simulink model "DreiTankSim_Visual"  (R2021a)
settings: Solver=ode5  StartTime=0.0  StopTime=inf  RelTol=1e-3
model workspace (MAT data in the model file):
  A1 = 20
  A2 = 20
  A3 = 20
  Kt = 1
  Kv = 8.75529661017
  Kvgekop = 6.21621117085
  k1 = 1.5
  k2 = 1.5
  k3 = 1.5
  k4 = 5
  k5 = 5
  k6 = 5
libraries: pid_lib x3, sldrtlib x3
(part 1 of 2)
settings Model: Creator=Ogulcan  LastModifiedBy=Ogulcan
settings RTWCC: Description=Simulink Desktop Real-Time  SystemTargetFile=sldrt.tlc  TemplateMakefile=sldrt.tmf  RTWCompilerOptimization=on
settings CodeAppCC: MaxIdLength=95
settings SimulinkDesktopRealTimeCC: TargetPreCompLibLocation=E:\MathWorks\r2021a\toolbox\sldrt\lib\win64

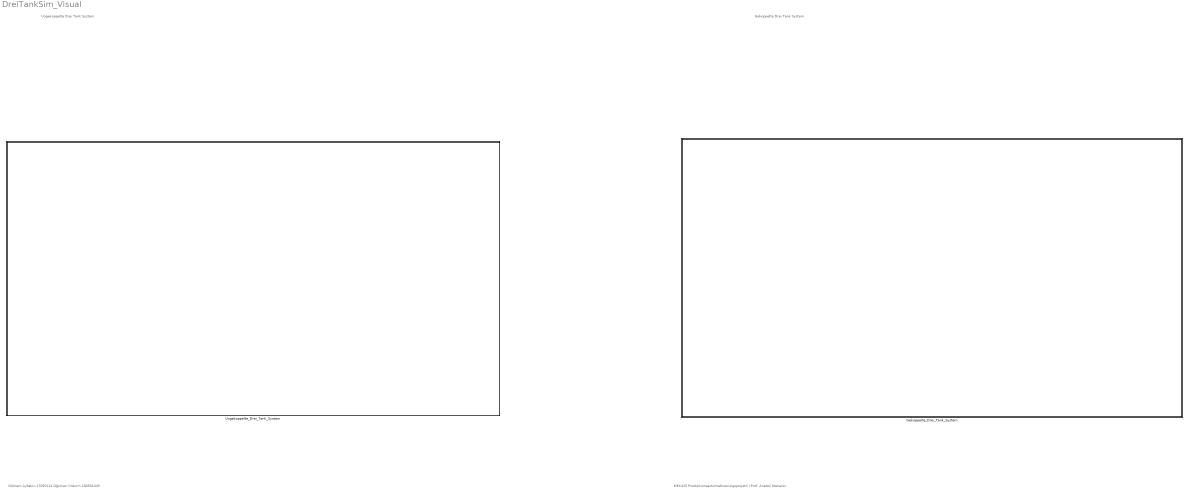
== system DreiTankSim_Visual ==
  note: Görkem Aytekin 17050114
      | Oğulcan Yıldırım 180501045
  note: Ungekoppelte Drei Tank System
  note: Gekoppelte Drei Tank System
  note: MEC425 Produktionsautomatisierungsprojekt I Prof. Anatoli Makarov
  Gekoppelte_Drei_Tank_System : Subsystem
      mask Display: image('C:\Users\Oğulcan\OneDrive\Masaüstü\GörOgiProjekt\MatlabGUİ\GuiTemiz\GekoppeltSim.png'); % Use "Edit Image" on toolstrip to change.
  Ungekoppelte_Drei_Tank_System : Subsystem
      mask Display: image('C:\Users\Oğulcan\OneDrive\Masaüstü\GörOgiProjekt\MatlabGUİ\GuiTemiz\ungekoppeltFotoSim.png'); % Use "Edit Image" on toolstrip to change.

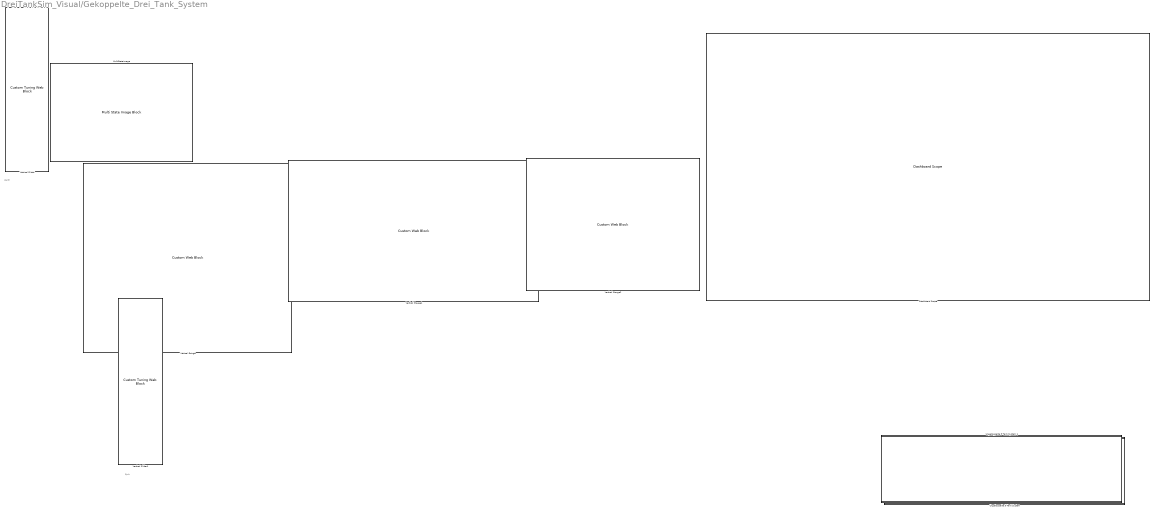
== system DreiTankSim_Visual/Gekoppelte_Drei_Tank_System ==
  note: Quit
  note: Ventil
  Dashboard Scope : DashboardScope  Ymin=0  Ymax=5000  LegendPosition=Right
  MultiStateImage : MultiStateImageBlock  ScaleMode=Fill
  "Ungekoppelte 3 Tank System " : Subsystem
      mask Display: image('C:\Users\Oğulcan\OneDrive\Masaüstü\GörOgiProjekt\MatlabGUİ\GuiTemiz\Taulogo.png'); % Use "Edit Image" on toolstrip to change.
  Ungekoppelte 3 Tank System 1 : Subsystem
      mask Display: image('C:\Users\Oğulcan\OneDrive\Masaüstü\GörOgiProjekt\MatlabGUİ\GuiTemiz\Taulogo.png'); % Use "Edit Image" on toolstrip to change.
  Vertical Gauge : CustomWebBlock  LabelPosition=Hide  ShowInitialText=on  Configuration="{\"components\":[{\"name\":\"LinearScaleComponent\",\"settings\":{\"bounds\":{\"max\":5000,\"min\":0,\"tickInterval\":500},\"internalTickHeightScaleFactor\":0.5,\"labelColor\":[0,255,0],\"labelFont\":{\"font\":\"Arial\",\"fontSize\":12},\"labelTransparency\":0.5,\"needleImage\":{\"size\":[21,75],\"src\":\"data:image\\/svg+xml;base64,PHN2ZyB4bWxucz0iaHR0cDovL3d3dy53My5vcmcvMjAwMC9zdmciIHhtbG5zOnhsaW5rPSJodHRwOi8vd3d3LnczLm9yZy8xOTk5L3hsaW5rIiB2aWV3Qm94PSIwIDAgMjEgNzUiPjxkZWZzPjxzdHlsZT4uY2xzLTF7ZmlsbDpub25lO30uY2xzLTJ7aXNvbGF0aW9uOmlzb2xhdGU7fS5jbHMtM3tjbGlwLXBhdGg6dXJsKCNjbGlwLXBhdGgpO30uY2xzLTR7b3BhY2l0eTowLjM7bWl4LWJsZW5kLW1vZGU6bXVsdGlwbHk7fS5jbHMtNXtmaWxsOiNlYjI2Mjk7fTwvc3R5bGU+PGNsaXBQYXRoIGlkPSJjbGlwLXBhdGgiIHRyYW5zZm9y ...(+1928 chars)\",\"srcOrientation\":\"horizontal\"},\"needleOffset\":[-0.01094391244870041,0],\"needleSize\":{\"height\":0.06,\"width\":0.48},\"position\":[-0.022724338282763074,0.21281719924812031,0.4357377819548872,0.6807617817947063],\"scaleColors\":[],\"scaleColorsSize\":0.2,\"showLabels\":1,\"showMinorTicks\":0,\"showSpanLine\":1,\"showTicks\":1,\"tickColor\":[204,204,204],\"tickTransparency\":0.5,\"valueBarColor\":[127,205,255],\"valueBarOffset\":-0.01,\"valueBarSize\":0.92,\"valueBarTransparency\":1}},{\"name\":\"BackgroundImageComponent\",\"settings\":{\"image\":{\"size\":[293,266],\"src\":\"data:image\\/png;base64,iVBORw0KGgoAAAANSUhEUgAAASUAAAEKCAYAAABUnUOUAAAACXBIWXMAABJ0AAASdAHeZh94AAANmUlEQVR4Xu3djVLbWBIGUP8Qktr3f9cEMPbeNhYjPBDEYMzt24eq1CSzxHSfT\\/6Qxay1WvmYBPbtN4f2a79er4\\/\\/RDOWwH4f0a4fp5xn\\/xxr0eTbbJLP\\/+nx40A9e5DzP3\\/6a3iAPgQ2m018s5k+5NxHLP+aonwpdZqLsb5I4HA4KKMvsr3Uw5YvpbPvnpdy9TiJBF45W040\\/Xijli+liNRBOd6B\\/dpGcs6Rs1LKkZMpLyDw1ks3L+kugHvBh1BKF8T0UAQIfF5AKX3e0CMQIHBBAaXUMF3svuAR1fFDxX9\\/dvpv0F ...(+4502 chars)\",\"srcOrientation\":\"vertical\"},\"position\":[0,0,1,1],\"scaleMode\":\"0\"}},{\"name\":\"ForegroundImageComponent\",\"settings\":{\"image\":{\"size\":[0,0],\"src\":\"default\",\"srcOrientation\":[]},\"isForeground\":1,\"position\":[0,0,1,1],\"scaleMode\":\"0\"}}],\"settings\":{\"BindingType\":\"signal\",\"backgroundColor\":[255,255,255,\"1\"],\"backgroundOffset\":0,\"backgroundOpacity\":0,\"fixedAspectRatio\":\"on\",\"orientation\":\"vertical\",\"showBackgroundColor\":false,\"value\":0},\"type\":\"LinearGauge\"}"
  Vertical Gauge1 : CustomWebBlock  LabelPosition=Hide  ShowInitialText=on  Configuration="{\"components\":[{\"name\":\"LinearScaleComponent\",\"settings\":{\"bounds\":{\"max\":5000,\"min\":0,\"tickInterval\":500},\"internalTickHeightScaleFactor\":0.5,\"labelColor\":[0,255,0],\"labelFont\":{\"font\":\"Arial\",\"fontSize\":12},\"labelTransparency\":0.5,\"needleImage\":{\"size\":[21,75],\"src\":\"data:image\\/svg+xml;base64,PHN2ZyB4bWxucz0iaHR0cDovL3d3dy53My5vcmcvMjAwMC9zdmciIHhtbG5zOnhsaW5rPSJodHRwOi8vd3d3LnczLm9yZy8xOTk5L3hsaW5rIiB2aWV3Qm94PSIwIDAgMjEgNzUiPjxkZWZzPjxzdHlsZT4uY2xzLTF7ZmlsbDpub25lO30uY2xzLTJ7aXNvbGF0aW9uOmlzb2xhdGU7fS5jbHMtM3tjbGlwLXBhdGg6dXJsKCNjbGlwLXBhdGgpO30uY2xzLTR7b3BhY2l0eTowLjM7bWl4LWJsZW5kLW1vZGU6bXVsdGlwbHk7fS5jbHMtNXtmaWxsOiNlYjI2Mjk7fTwvc3R5bGU+PGNsaXBQYXRoIGlkPSJjbGlwLXBhdGgiIHRyYW5zZm9y ...(+1928 chars)\",\"srcOrientation\":\"horizontal\"},\"needleOffset\":[-0.01094391244870041,0],\"needleSize\":{\"height\":0.06,\"width\":0.38},\"position\":[-0.05307664627563872,0.23195564516129033,0.3876008064516129,0.9625764663548039],\"scaleColors\":[],\"scaleColorsSize\":0.2,\"showLabels\":1,\"showMinorTicks\":0,\"showSpanLine\":1,\"showTicks\":1,\"tickColor\":[204,204,204],\"tickTransparency\":0.5,\"valueBarColor\":[127,205,255],\"valueBarOffset\":-0.03,\"valueBarSize\":0.92,\"valueBarTransparency\":1}},{\"name\":\"BackgroundImageComponent\",\"settings\":{\"image\":{\"size\":[313,175],\"src\":\"data:image\\/png;base64,iVBORw0KGgoAAAANSUhEUgAAATkAAACvCAYAAACGqakbAAAACXBIWXMAABJ0AAASdAHeZh94AAAG3ElEQVR4Xu3dwXIbRwwFwCiV\\/\\/\\/gHKyYPim0E3mWGDyspnVTFQfANshHSjLptz98rQq8Px14fP\\/nahG3jwt8+z7B24cp7DG+kj0DeHC+7vrxgfJ6NRUIECgVEHKlnIrdSOD5ycmT1Y2WtzKqkFvRctuvLPD8a4ivfK1HXZuQO2rdLpbAeQJC7rydu2ICRwkIuaPW7WIJnCcg5M7buSsmcJSAkDtq3S6WwHkCQu68nbtiAkcJCLmj1u1iCZwnIOTO27krJnCUgJB7fd3+EenrhioQ2CYg5LbRKkyAwAQBITdhC2YgQGCbgJDbRqvw ...(+2096 chars)\",\"srcOrientation\":\"vertical\"},\"position\":[0,0,1,1],\"scaleMode\":\"0\"}},{\"name\":\"ForegroundImageComponent\",\"settings\":{\"image\":{\"size\":[0,0],\"src\":\"default\",\"srcOrientation\":[]},\"isForeground\":1,\"position\":[0,0,1,1],\"scaleMode\":\"0\"}}],\"settings\":{\"BindingType\":\"signal\",\"backgroundColor\":[255,255,255,\"1\"],\"backgroundOffset\":0,\"backgroundOpacity\":0,\"fixedAspectRatio\":\"on\",\"orientation\":\"vertical\",\"showBackgroundColor\":false,\"value\":0},\"type\":\"LinearGauge\"}"
  Vertical Gauge2 : CustomWebBlock  LabelPosition=Hide  ShowInitialText=on  Configuration="{\"components\":[{\"name\":\"LinearScaleComponent\",\"settings\":{\"bounds\":{\"max\":5000,\"min\":0,\"tickInterval\":500},\"internalTickHeightScaleFactor\":0.5,\"labelColor\":[0,255,0],\"labelFont\":{\"font\":\"Arial\",\"fontSize\":12},\"labelTransparency\":0.5,\"needleImage\":{\"size\":[21,75],\"src\":\"data:image\\/svg+xml;base64,PHN2ZyB4bWxucz0iaHR0cDovL3d3dy53My5vcmcvMjAwMC9zdmciIHhtbG5zOnhsaW5rPSJodHRwOi8vd3d3LnczLm9yZy8xOTk5L3hsaW5rIiB2aWV3Qm94PSIwIDAgMjEgNzUiPjxkZWZzPjxzdHlsZT4uY2xzLTF7ZmlsbDpub25lO30uY2xzLTJ7aXNvbGF0aW9uOmlzb2xhdGU7fS5jbHMtM3tjbGlwLXBhdGg6dXJsKCNjbGlwLXBhdGgpO30uY2xzLTR7b3BhY2l0eTowLjM7bWl4LWJsZW5kLW1vZGU6bXVsdGlwbHk7fS5jbHMtNXtmaWxsOiNlYjI2Mjk7fTwvc3R5bGU+PGNsaXBQYXRoIGlkPSJjbGlwLXBhdGgiIHRyYW5zZm9y ...(+1928 chars)\",\"srcOrientation\":\"horizontal\"},\"needleOffset\":[-0.01094391244870041,0],\"needleSize\":{\"height\":0.06,\"width\":0.48},\"position\":[0.003223915592028136,0.4366930751173709,0.5352112676056338,0.9722547870261821],\"scaleColors\":[],\"scaleColorsSize\":0.2,\"showLabels\":1,\"showMinorTicks\":0,\"showSpanLine\":1,\"showTicks\":1,\"tickColor\":[204,204,204],\"tickTransparency\":0.5,\"valueBarColor\":[127,205,255],\"valueBarOffset\":-0.01,\"valueBarSize\":0.91,\"valueBarTransparency\":1}},{\"name\":\"BackgroundImageComponent\",\"settings\":{\"image\":{\"size\":[235,176],\"src\":\"data:image\\/png;base64,iVBORw0KGgoAAAANSUhEUgAAAOsAAACwCAYAAADuQ5nhAAAG4klEQVR4Xu3d7U5aWwAGYfmw3v\\/F+kMpcNaiajytRa2V4vCQGKNR2e8M44Ym3V5duSGAAAIIIIAAAggggAACCCCAAAIfILDb7Rbz7QM\\/wrd+DQK75XL5fRzq7mscrqP8H4HNZjP8LTdT4GKxmCLdmgS2D5Huh+f5Nj92+0oEZqir1WrG+iiQxK8k8A3Hut1ul4+hrtfr\\/XTt7PoGcGf4JfMp0f7m5uYg0W\\/cMzT0dw5pPnN6DHX\\/8HT46Sd7DfR3IH\\/2T5mxPnc1hc7fxG4tAkc9E96SbU2YgFjDck1rERBry6c1YQJiDcs1rUVArC2f1oQJiDUs17QWAbG2fFoT ...(+2100 chars)\",\"srcOrientation\":\"vertical\"},\"position\":[0,0,1,1],\"scaleMode\":\"0\"}},{\"name\":\"ForegroundImageComponent\",\"settings\":{\"image\":{\"size\":[0,0],\"src\":\"default\",\"srcOrientation\":[]},\"isForeground\":1,\"position\":[0,0,1,1],\"scaleMode\":\"0\"}}],\"settings\":{\"BindingType\":\"signal\",\"backgroundColor\":[255,255,255,\"1\"],\"backgroundOffset\":0,\"backgroundOpacity\":0,\"fixedAspectRatio\":\"on\",\"orientation\":\"vertical\",\"showBackgroundColor\":false,\"value\":0},\"type\":\"LinearGauge\"}"
  Vertical Slider : CustomTuningWebBlock  LabelPosition=Hide  ShowInitialText=on  Configuration="{\"components\":[{\"name\":\"LinearScaleComponent\",\"settings\":{\"bounds\":{\"max\":10,\"min\":0,\"tickInterval\":\"auto\"},\"internalTickHeightScaleFactor\":1,\"labelColor\":[255,255,0],\"labelFont\":{\"font\":\"Arial\",\"fontSize\":12},\"labelOffset\":0.05,\"labelTransparency\":1,\"needleImage\":{\"size\":[842,596],\"src\":\"data:image\\/svg+xml;base64,PD94bWwgdmVyc2lvbj0iMS4wIiBlbmNvZGluZz0idXRmLTgiPz4NCjwhLS0gR2VuZXJhdG9yOiBBZG9iZSBJbGx1c3RyYXRvciAyNS4wLjAsIFNWRyBFeHBvcnQgUGx1Zy1JbiAuIFNWRyBWZXJzaW9uOiA2LjAwIEJ1aWxkIDApICAtLT4NCjxzdmcgdmVyc2lvbj0iMS4xIg0KCSBpZD0ic3ZnOCIgeG1sbnM6Y2M9Imh0dHA6Ly9jcmVhdGl2ZWNvbW1vbnMub3JnL25zIyIgeG1sbnM6ZGM9Imh0dHA6Ly9wdXJsLm9yZy9kYy9lbGVtZW50cy8xLjEvIiB4bWxuczppbmtzY2FwZT0iaHR0cDovL3d3dy5pbmtzY2FwZS5vcmcvbmFtZXNw ...(+2376 chars)\",\"srcOrientation\":\"vertical\"},\"needleOffset\":[0.02,-0.8],\"needleSize\":{\"height\":0.07532387955182072,\"width\":0.43386243386243384},\"position\":[0.027412280701754384,0.2830188679245283,0.5832841981132075,0.9524201127819549],\"scaleColors\":[],\"scaleColorsSize\":0.2,\"showLabels\":1,\"showMinorTicks\":0,\"showSpanLine\":1,\"showTicks\":1,\"tickColor\":[234,234,234],\"tickTransparency\":1,\"valueBarColor\":[0,255,255],\"valueBarOffset\":-0.28,\"valueBarSize\":0.1,\"valueBarTransparency\":1}},{\"name\":\"BackgroundImageComponent\",\"settings\":{\"image\":{\"size\":[101,380],\"src\":\"data:image\\/svg+xml;base64,PD94bWwgdmVyc2lvbj0iMS4wIiBlbmNvZGluZz0iVVRGLTgiIHN0YW5kYWxvbmU9Im5vIj8+CjxzdmcKICAgeG1sbnM6ZGM9Imh0dHA6Ly9wdXJsLm9yZy9kYy9lbGVtZW50cy8xLjEvIgogICB4bWxuczpjYz0iaHR0cDovL2NyZWF0aXZlY29tbW9ucy5vcmcvbnMjIgogICB4bWxuczpyZGY9Imh0dHA6Ly93d3cudzMub3JnLzE5OTkvMDIvMjItcmRmLXN5bnRheC1ucyMiCiAgIHhtbG5zOnN2Zz0iaHR0cDovL3d3dy53My5vcmcvMjAwMC9zdmciCiAgIHhtbG5zPSJodHRwOi8vd3d3LnczLm9yZy8yMDAwL3N2ZyIKICAgeG1sbnM6 ...(+3116 chars)\",\"srcOrientation\":\"vertical\"},\"position\":[0,0,1,1],\"scaleMode\":\"0\"}},{\"name\":\"ForegroundImageComponent\",\"settings\":{\"image\":{\"size\":[0,0],\"src\":\"default\",\"srcOrientation\":[]},\"isForeground\":1,\"position\":[0,0,1,1],\"scaleMode\":\"0\"}}],\"settings\":{\"BindingType\":\"param\",\"aspectRatio\":0.2651006711409396,\"backgroundColor\":[0,0,0,\"1\"],\"backgroundOffset\":0,\"backgroundOpacity\":1,\"fixedAspectRatio\":\"on\",\"orientation\":\"vertical\",\"showBackgroundColor\":false,\"value\":0},\"type\":\"LinearGauge\"}"
  Vertical Slider1 : CustomTuningWebBlock  LabelPosition=Hide  ShowInitialText=on  Configuration="{\"components\":[{\"name\":\"LinearScaleComponent\",\"settings\":{\"bounds\":{\"max\":2,\"min\":0,\"tickInterval\":\"auto\"},\"internalTickHeightScaleFactor\":1,\"labelColor\":[255,255,0],\"labelFont\":{\"font\":\"Arial\",\"fontSize\":12},\"labelOffset\":0.05,\"labelTransparency\":1,\"needleImage\":{\"size\":[842,596],\"src\":\"data:image\\/svg+xml;base64,PD94bWwgdmVyc2lvbj0iMS4wIiBlbmNvZGluZz0idXRmLTgiPz4NCjwhLS0gR2VuZXJhdG9yOiBBZG9iZSBJbGx1c3RyYXRvciAyNS4wLjAsIFNWRyBFeHBvcnQgUGx1Zy1JbiAuIFNWRyBWZXJzaW9uOiA2LjAwIEJ1aWxkIDApICAtLT4NCjxzdmcgdmVyc2lvbj0iMS4xIg0KCSBpZD0ic3ZnOCIgeG1sbnM6Y2M9Imh0dHA6Ly9jcmVhdGl2ZWNvbW1vbnMub3JnL25zIyIgeG1sbnM6ZGM9Imh0dHA6Ly9wdXJsLm9yZy9kYy9lbGVtZW50cy8xLjEvIiB4bWxuczppbmtzY2FwZT0iaHR0cDovL3d3dy5pbmtzY2FwZS5vcmcvbmFtZXNw ...(+2376 chars)\",\"srcOrientation\":\"vertical\"},\"needleOffset\":[0.02,-0.8],\"needleSize\":{\"height\":0.07532387955182072,\"width\":0.43386243386243384},\"position\":[0.027412280701754384,0.2830188679245283,0.5832841981132075,0.9524201127819549],\"scaleColors\":[],\"scaleColorsSize\":0.2,\"showLabels\":1,\"showMinorTicks\":0,\"showSpanLine\":1,\"showTicks\":1,\"tickColor\":[234,234,234],\"tickTransparency\":1,\"valueBarColor\":[0,255,255],\"valueBarOffset\":-0.28,\"valueBarSize\":0.1,\"valueBarTransparency\":1}},{\"name\":\"BackgroundImageComponent\",\"settings\":{\"image\":{\"size\":[101,380],\"src\":\"data:image\\/svg+xml;base64,PD94bWwgdmVyc2lvbj0iMS4wIiBlbmNvZGluZz0iVVRGLTgiIHN0YW5kYWxvbmU9Im5vIj8+CjxzdmcKICAgeG1sbnM6ZGM9Imh0dHA6Ly9wdXJsLm9yZy9kYy9lbGVtZW50cy8xLjEvIgogICB4bWxuczpjYz0iaHR0cDovL2NyZWF0aXZlY29tbW9ucy5vcmcvbnMjIgogICB4bWxuczpyZGY9Imh0dHA6Ly93d3cudzMub3JnLzE5OTkvMDIvMjItcmRmLXN5bnRheC1ucyMiCiAgIHhtbG5zOnN2Zz0iaHR0cDovL3d3dy53My5vcmcvMjAwMC9zdmciCiAgIHhtbG5zPSJodHRwOi8vd3d3LnczLm9yZy8yMDAwL3N2ZyIKICAgeG1sbnM6 ...(+3116 chars)\",\"srcOrientation\":\"vertical\"},\"position\":[0,0,1,1],\"scaleMode\":\"0\"}},{\"name\":\"ForegroundImageComponent\",\"settings\":{\"image\":{\"size\":[0,0],\"src\":\"default\",\"srcOrientation\":[]},\"isForeground\":1,\"position\":[0,0,1,1],\"scaleMode\":\"0\"}}],\"settings\":{\"BindingType\":\"param\",\"aspectRatio\":0.2651006711409396,\"backgroundColor\":[0,0,0,\"1\"],\"backgroundOffset\":0,\"backgroundOpacity\":1,\"fixedAspectRatio\":\"on\",\"orientation\":\"vertical\",\"showBackgroundColor\":false,\"value\":0},\"type\":\"LinearGauge\"}"
